simulink model "MCC"  (R2017b)
settings: Solver=ode15s  StartTime=0.0  StopTime=0.2  RelTol=1e-3
InitFcn:
  | MCC_constants
values from neighbouring files (symbols this model uses):
  b = 3.5077E-6    (= 3.5077e-06)    [MCC_constants.m]
  Cr = 0    [MCC_constants.m]
  J = 3.2284E-6    (= 3.2284e-06)    [MCC_constants.m]
  K = 0.0274    [MCC_constants.m]
  L = 2.75E-6    (= 2.75e-06)    [MCC_constants.m]
  R = 4    [MCC_constants.m]
settings Model: Creator=TABLE 6  LastModifiedBy=TABLE 6

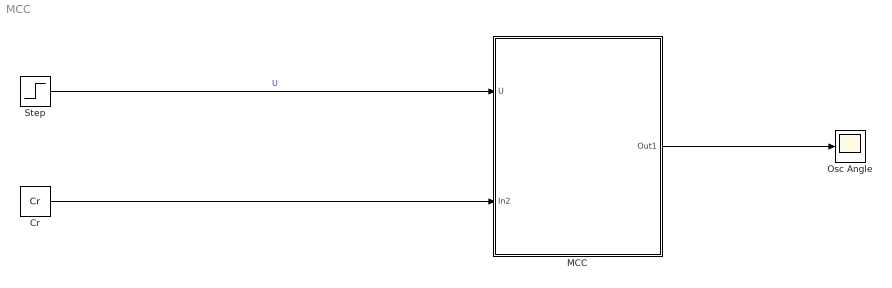
== system MCC ==
  Cr : Constant  Value=Cr
  MCC : Subsystem
  Osc Angle : Scope
  Step : Step  Time=0  After=12  SampleTime=0
  wires:
  Step/1 -> MCC/1(U)  "U"
  Cr/1 -> MCC/2(In2)
  MCC/1(Out1) -> Osc Angle/1

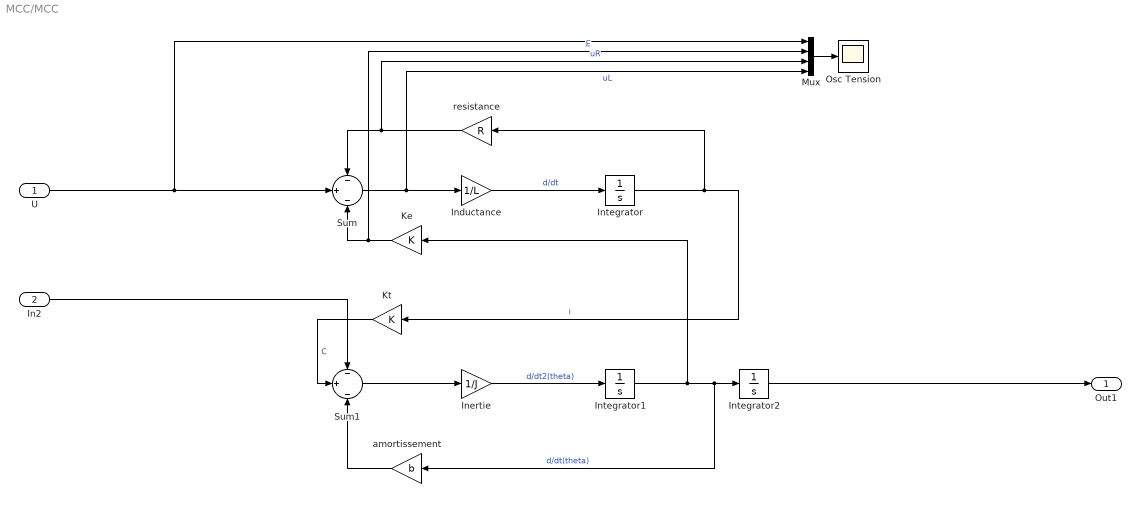
== system MCC/MCC ==
  U : Inport
  In2 : Inport  Port=2
  Inductance : Gain  Gain=1/L
  Inertie : Gain  Gain=1/J
  Integrator : Integrator
  Integrator1 : Integrator
  Integrator2 : Integrator
  Ke : Gain  Gain=K
  Kt : Gain  Gain=K
  Mux : Mux
  Osc Tension : Scope
  Sum : Sum  Inputs=-|+|-
  Sum1 : Sum  Inputs=-|+|-
  amortissement : Gain  Gain=b
  resistance : Gain  Gain=R
  Out1 : Outport
  wires:
  resistance/1 -> Mux/3, Sum/1  "uR"
  Sum/1 -> Mux/4, Inductance/1  "uL"
  Inductance/1 -> Integrator/1  "d/dt"
  Inertie/1 -> Integrator1/1  "d/dt2(theta)"
  Sum1/1 -> Inertie/1
  Mux/1 -> Osc Tension/1
  Integrator1/1 -> Ke/1, amortissement/1, Integrator2/1  "d/dt(theta)"
  U/1 -> Mux/1, Sum/2
  Integrator2/1 -> Out1/1
  Integrator/1 -> resistance/1, Kt/1  "i"
  In2/1 -> Sum1/1
  amortissement/1 -> Sum1/3
  Ke/1 -> Mux/2, Sum/3  "E"
  Kt/1 -> Sum1/2  "C"
